simulink model "CBCVacc"  (Simulink 7.5)
settings: Solver=ode4  StartTime=0.0  StopTime=Inf  FixedStep=0.001  RelTol=1e-3
PostLoadFcn:
  | , if any(exist('dsrtsu_mdlpostloadfcn', 'file') == [2, 3, 6]), try dsrtsu_mdlpostloadfcn('Execute', bdroot); catch fprintf('Error in PostLoadFcn (dsrtsu_mdlpostloadfcn) for model "%s":\n %s\n', bdroot, lasterr); end, end,
libraries: simulink x5, rtilib1104 x3, dsparch4 x2
settings Model: DSRTSU_INTERNAL_RTI_VER=380  DSRTSU_INTERNAL_RTI_TYPE=rti1104  Creator=user  LastModifiedBy=user  BufferReuse=off
settings OptimizationCC: BlockReduction=off  ConditionallyExecuteInputs=off  OptimizeBlockIOStorage=off  BufferReuse=off  ExpressionFolding=off  LocalBlockOutputs=off  InitFltsAndDblsToZero=on
settings DebuggingCC: SaveWithParameterizedLinksMsg=none  StrictBusMsg=Warning
settings HardwareCC: ProdIntDivRoundTo=Zero  ProdEndianess=BigEndian  ProdHWDeviceType=Generic->Custom  TargetIntDivRoundTo=Zero  TargetEndianess=BigEndian  TargetHWDeviceType=Generic->Custom
settings RTWCC: SystemTargetFile=rti1104.tlc  MakeCommand=make_rti  TemplateMakefile=rti1104.tmf  Description=dSPACE DS1104 Hardware Platform  ProcessScript=rti1104_make_rtw_hook
settings STFCustomTargetCC: TargetFcnLib=ansi_tfl_tmw.mat  ParMdlRefBuildCompliant=on  GeneratePreprocessorConditionals=Disable all  SystemTargetFile=rti1104.tlc
settings GRTTargetCC: TargetFcnLib=ansi_tfl_tmw.mat  CompOptLevelCompliant=off  MatFileLogging=off  ExtModeMexFile=noextcomm
settings CustomProperty: DataType=RTWOptions_EnumType_C__DSpace_matlab_rti1104_tlc_rti1104_1InitialSimState  Value=RUN
settings EnumStrPairs: String=RUN

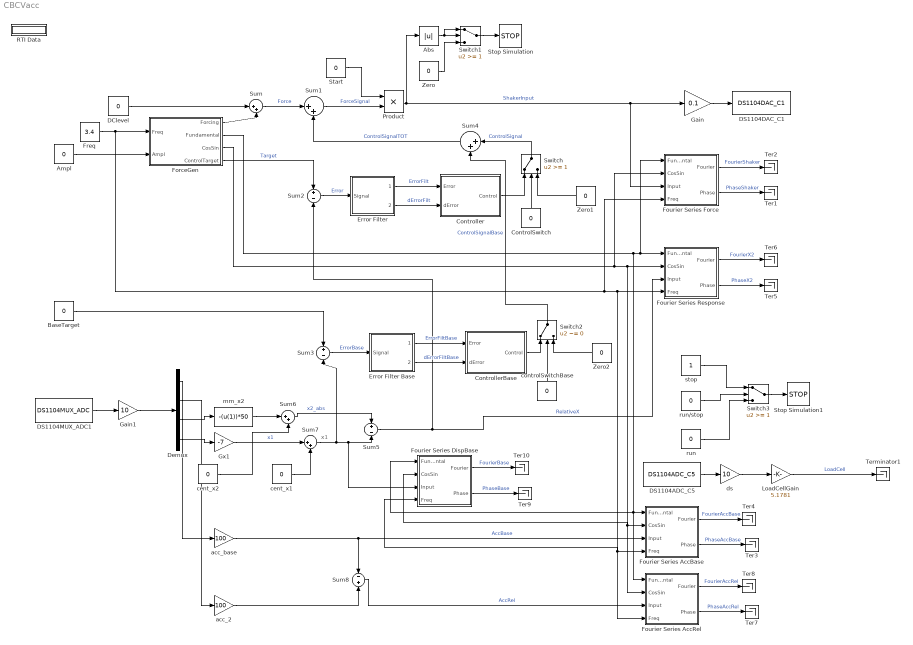
== system CBCVacc ==
  note: x1
  Abs : Abs
  Ampl : Constant  Value=0
  BaseTarget : Constant  Value=0  OutDataType=sfix(16)  OutScaling=2^0
  ControlSwitch : Constant  Value=0  OutDataType=sfix(16)  OutScaling=2^0
  Controller : Subsystem
  ControllerBase : Subsystem
  DClevel : Constant  Value=0  OutDataType=sfix(16)  OutScaling=2^0
  DS1104ADC_C5 : rtilib1104/DS1104 MASTER PPC/DS1104ADC_C5  SystemSampleTime=-1  ChannelNo=5  TriggerMode=0  Reserved1=[]  Reserved2=[]  Reserved3=[]  Reserved4=[]  DialogFcn=gui1104adc  UnitName={ 'DS1104ADC_C' }  UnitValues={ 5 }  DSProperties=struct('RTI',struct('Version',uint32(1),'BlockType',struct('isSLSource',uint8(1),'isSLSink',uint8(0),'isHWSource',uint8(1),'isHWSink',uint8(0),'isSetup',uint8(0),'isInline',uint8(1),'isNonInline',uint8(0),'isInterrupt',uint8(0),'isChannelwise',uint8(1)),'IOBoardType','DS1104MASTER','UnitType','ADC','Identifier','ADC','DialogType','ML','BlockSet','NONE','SlaveProcessor','NONE'))
  DS1104DAC_C1 : rtilib1104/DS1104 MASTER PPC/DS1104DAC_C1  SystemSampleTime=-1  ChannelNo=1  InitValue=0  TermMode=0  TermValue=0  Reserved1=[]  Reserved2=[]  Reserved3=[]  Reserved4=[]  DialogFcn=gui1104dac  UnitName={ 'DS1104DAC_C'}  UnitValues={ 1 }  DSProperties=struct('RTI',struct('Version',uint32(1),'BlockType',struct('isSLSource',uint8(0),'isSLSink',uint8(1),'isHWSource',uint8(0),'isHWSink',uint8(1),'isSetup',uint8(0),'isInline',uint8(1),'isNonInline',uint8(0),'isInterrupt',uint8(0),'isChannelwise',uint8(1)),'IOBoardType','DS1104MASTER','UnitType','DAC','Identifier','DAC','DialogType','ML','BlockSet','NONE','SlaveProcessor','NONE'))
  DS1104MUX_ADC1 : rtilib1104/DS1104 MASTER PPC/DS1104MUX_ADC  SystemSampleTime=-1  ChannelNos=[1 2 3 4]  TriggerMode=0  Reserved1=[]  Reserved2=[]  Reserved3=[]  Reserved4=[]  DialogFcn=gui1104mux_adc  UnitName={ 'DS1104MUX_ADC' }  UnitValues={ [] }  DSProperties=struct('RTI',struct('Version',uint32(1),'BlockType',struct('isSLSource',uint8(1),'isSLSink',uint8(0),'isHWSource',uint8(1),'isHWSink',uint8(0),'isSetup',uint8(0),'isInline',uint8(1),'isNonInline',uint8(0),'isInterrupt',uint8(0),'isChannelwise',uint8(0)),'IOBoardType','DS1104MASTER','UnitType','ADC','Identifier','ADCMUX','DialogType','ML','BlockSet','NONE','SlaveProcessor','NONE'))
  Demux : Demux
  Error Filter : Subsystem
  Error Filter Base : Subsystem
  ForceGen : Subsystem
  Fourier Series AccBase : Subsystem
  Fourier Series AccRel : Subsystem
  Fourier Series DispBase : Subsystem
  Fourier Series Force : Subsystem
  Fourier Series Response : Subsystem
  Freq : Constant  Value=3.4  SampleTime=-1
  Gain : Gain  Gain=0.1
  Gain1 : Gain  Gain=10  ParameterDataType=sfix(16)  ParameterScaling=2^0  OutDataType=sfix(16)  OutScaling=2^0
  Gx1 : Gain  Gain=-7  ParameterDataType=fixdt(1, 16)  ParameterScaling=2^0  OutDataType=fixdt(1, 16)  OutScaling=2^0
  LoadCellGain : Gain  Gain=5.1781  ParameterDataType=fixdt(1, 16)  ParameterScaling=2^0  OutDataType=fixdt(1, 16)  OutScaling=2^0
  Product : Product  OutDataType=sfix(16)  OutScaling=2^0  RndMeth=Zero
  RTI Data : Subsystem  Tag=struct('RTIDataServer',struct('RTIDataServerVs','2','RTIModelDescription','struct(''main'',''CBCVacc'',''sub'','''',''isMp'',0)'))  LoadFcn="if exist('rtidc'), try,  rtidc('DataHostBlockClbLoad', gcbh); catch, disp(['Warning: ''LoadFcn'' for RTI Data block failed: ' lasterr]); end, end,"
      settings: CopyFcn="if exist('rtidc'), try,  rtidc('DataHostBlockClbCopy', gcbh); catch, disp(['Warning: ''CopyFcn'' for RTI Data block failed: ' lasterr]); end, end,"  DeleteFcn="if exist('rtidc'), try,  rtidc('DataHostBlockClbDelete', gcbh); catch, disp(['Warning: ''DeleteFcn'' for RTI Data block failed: ' lasterr]); end, end,"  ModelCloseFcn="if exist('rtidc'), try,  rtidc('DataHostBlockClbModelClose', gcbh); catch, disp(['Warning: ''ModelCloseFcn'' for RTI Data block failed: ' lasterr]); end, end,"  PreSaveFcn="if exist('rtidc'), try,  rtidc('DataHostBlockClbPreSave', gcbh); catch, disp(['Warning: ''PreSaveFcn'' for RTI Data block failed: ' lasterr]); end, end,"  PostSaveFcn="if exist('rtidc'), try,  rtidc('DataHostBlockClbPostSave', gcbh); catch, disp(['Warning: ''PostSaveFcn'' for RTI Data block failed: ' lasterr]); end, end,"  NameChangeFcn="if exist('rtidc'), try,  rtidc('DataHostBlockClbNameChange', gcbh); catch, disp(['Warning: ''NameChangeFcn'' for RTI Data block failed: ' lasterr]); end, end,"
      mask Type: RTI_DATA_HOST
      mask Description:
      | RTI Data Block.
      | This block is used by RTI to store internal model-dependent data.
      | Please keep this block on the root level of the model. Deleting this block will result in data loss.
      | 
      | NEVER DELETE OR COPY THIS BLOCK!
      mask Help:
      | RTI Data Block.
      | This block is used by RTI to store internal model-dependent data.
      | Please keep this block on the root level of the model. Deleting this block will result in data loss.
      | 
      | NEVER DELETE OR COPY THIS BLOCK!
      mask Display:
      | text(0.5, 0.5, 'RTI Data', 'HorizontalAlignment', 'center');
      | plot([1 0]);
  Start : Constant  Value=0  OutDataType=sfix(16)  OutScaling=2^0
  Stop Simulation : Stop
  Stop Simulation1 : Stop
  Sum : Sum  Inputs=|++  OutDataType=sfix(16)  OutScaling=2^0
  Sum1 : Sum  Inputs=|++
  Sum2 : Sum  Inputs=+|-
  Sum3 : Sum  Inputs=+|-
  Sum4 : Sum  Inputs=|++
  Sum5 : Sum  Inputs=+|-
  Sum6 : Sum  Inputs=|++  OutDataType=sfix(16)  OutScaling=2^0
  Sum7 : Sum  Inputs=|++  OutDataType=sfix(16)  OutScaling=2^0
  Sum8 : Sum  Inputs=-|+
  Switch : Switch  Threshold=1
  Switch1 : Switch  Threshold=1
  Switch2 : Switch  Criteria=u2 ~= 0
  Switch3 : Switch  Threshold=1
  Ter{1..10} (10 alike) : Terminator
  Terminator1 : Terminator
  Zero : Constant  Value=0  OutDataType=sfix(16)  OutScaling=2^0
  Zero1 : Constant  Value=0  OutDataType=sfix(16)  OutScaling=2^0
  Zero2 : Constant  Value=0  OutDataType=sfix(16)  OutScaling=2^0
  acc_2 : Gain  Gain=100  ParameterDataType=fixdt(1, 16)  ParameterScaling=2^0  OutDataType=fixdt(1, 16)  OutScaling=2^0
  acc_base : Gain  Gain=100  ParameterDataType=fixdt(1, 16)  ParameterScaling=2^0  OutDataType=fixdt(1, 16)  OutScaling=2^0
  cent_x1 : Constant  Value=0
  cent_x2 : Constant  Value=0
  controlSwitchBase : Constant  Value=0  OutDataType=sfix(16)  OutScaling=2^0
  ds : Gain  Gain=10  ParameterDataType=fixdt(1, 16)  ParameterScaling=2^0  OutDataType=fixdt(1, 16)  OutScaling=2^0
  mm_x2 : Fcn  Expr=-(u(1))*50
  run : Constant  Value=0  OutDataType=sfix(16)  OutScaling=2^0
  run/stop : Constant  Value=0  OutDataType=sfix(16)  OutScaling=2^0
  stop : Constant  OutDataType=sfix(16)  OutScaling=2^0
  wires:
  Freq/1 -> ForceGen/1(Freq), Fourier Series Force/4(Freq), Fourier Series Response/4(Freq), Fourier Series AccBase/4(Freq), Fourier Series AccRel/4(Freq), Fourier Series DispBase/4(Freq)
  Ampl/1 -> ForceGen/2(Ampl)
  ForceGen/3(CosSin) -> Fourier Series Force/2(CosSin), Fourier Series Response/2(CosSin), Fourier Series AccBase/2(CosSin), Fourier Series AccRel/2(CosSin), Fourier Series DispBase/2(CosSin)
  ForceGen/2(Fundamental) -> Fourier Series Response/1(Fundamental), Fourier Series Force/1(Fundamental), Fourier Series AccBase/1(Fundamental), Fourier Series AccRel/1(Fundamental), Fourier Series DispBase/1(Fundamental)
  Fourier Series Response/1(Fourier) -> Ter6/1  "FourierX2"
  Gain/1 -> DS1104DAC_C1/1
  Fourier Series Response/2(Phase) -> Ter5/1  "PhaseX2"
  ForceGen/1(Forcing) -> Sum/2
  DS1104MUX_ADC1/1 -> Gain1/1
  Gain1/1 -> Demux/1
  DClevel/1 -> Sum/1
  Switch1/1 -> Stop Simulation/1
  Abs/1 -> Switch1/2, Switch1/1
  Zero/1 -> Switch1/3
  Start/1 -> Product/1
  Sum/1 -> Sum1/1  "Force"
  Product/1 -> Abs/1, Gain/1, Fourier Series Force/3(Input)  "ShakerInput"
  Error Filter/1(Filtered) -> Controller/1(Error)  "ErrorFilt"
  Error Filter/2(dFiltered) -> Controller/2(dError)  "dErrorFilt"
  Sum2/1 -> Error Filter/1(Signal)  "Error"
  Controller/1(Control) -> Switch/1
  ControlSwitch/1 -> Switch/2
  Zero1/1 -> Switch/3
  ForceGen/4(ControlTarget) -> Sum2/1  "Target"
  Sum1/1 -> Product/2  "ForceSignal"
  Demux/1 -> acc_base/1
  Demux/3 -> mm_x2/1
  Demux/2 -> acc_2/1
  Demux/4 -> Gx1/1
  Error Filter Base/1(Filtered) -> ControllerBase/1(Error)  "ErrorFiltBase"
  Error Filter Base/2(dFiltered) -> ControllerBase/2(dError)  "dErrorFiltBase"
  ControllerBase/1(Control) -> Switch2/1
  Zero2/1 -> Switch2/3
  Sum3/1 -> Error Filter Base/1(Signal)  "ErrorBase"
  BaseTarget/1 -> Sum3/1
  Switch2/1 -> Sum4/2  "ControlSignalBase"
  Sum4/1 -> Sum1/2  "ControlSignalTOT"
  Switch/1 -> Sum4/1  "ControlSignal"
  Fourier Series Force/1(Fourier) -> Ter2/1  "FourierShaker"
  Fourier Series Force/2(Phase) -> Ter1/1  "PhaseShaker"
  Switch3/1 -> Stop Simulation1/1
  run/1 -> Switch3/3
  stop/1 -> Switch3/1
  run/stop/1 -> Switch3/2
  Sum5/1 -> Fourier Series Response/3(Input), Sum2/2  "RelativeX"
  controlSwitchBase/1 -> Switch2/2
  mm_x2/1 -> Sum6/1
  cent_x2/1 -> Sum6/2
  Sum6/1 -> Sum5/1  "x2_abs"
  Gx1/1 -> Sum7/1  "x1"
  cent_x1/1 -> Sum7/2
  Sum7/1 -> Sum3/2, Sum5/2, Fourier Series DispBase/3(Input)
  LoadCellGain/1 -> Terminator1/1  "LoadCell"
  acc_base/1 -> Fourier Series AccBase/3(Input), Sum8/1  "AccBase"
  DS1104ADC_C5/1 -> ds/1
  ds/1 -> LoadCellGain/1
  Fourier Series AccBase/1(Fourier) -> Ter4/1  "FourierAccBase"
  Fourier Series AccBase/2(Phase) -> Ter3/1  "PhaseAccBase"
  Fourier Series AccRel/1(Fourier) -> Ter8/1  "FourierAccRel"
  Fourier Series AccRel/2(Phase) -> Ter7/1  "PhaseAccRel"
  acc_2/1 -> Sum8/2
  Sum8/1 -> Fourier Series AccRel/3(Input)  "AccRel"
  Fourier Series DispBase/1(Fourier) -> Ter10/1  "FourierBase"
  Fourier Series DispBase/2(Phase) -> Ter9/1  "PhaseBase"

== system CBCVacc/Controller ==
  Error : Inport
  dError : Inport  Port=2
  Kd : Constant  Value=0
  Kp : Constant  Value=0
  Product : Product  RndMeth=Zero
  Product1 : Product  RndMeth=Zero
  Sum2 : Sum  Inputs=+|+
  Control : Outport
  wires:
  Kp/1 -> Product/1
  Kd/1 -> Product1/2
  Product/1 -> Sum2/1
  Product1/1 -> Sum2/2
  Error/1 -> Product/2
  Sum2/1 -> Control/1  "Control"
  dError/1 -> Product1/1

== system CBCVacc/ControllerBase ==
  Error : Inport
  dError : Inport  Port=2
  Kd : Constant  Value=0
  Kp : Constant  Value=0
  Product : Product  RndMeth=Zero
  Product1 : Product  RndMeth=Zero
  Sum2 : Sum  Inputs=+|+
  Control : Outport
  wires:
  Kp/1 -> Product/1
  Kd/1 -> Product1/2
  Product/1 -> Sum2/1
  Product1/1 -> Sum2/2
  Error/1 -> Product/2
  Sum2/1 -> Control/1  "Control"
  dError/1 -> Product1/1

== system CBCVacc/Error Filter ==
  Signal : Inport
  Analog Filter Design : dsparch4/Analog Filter Design  method=Butterworth  filttype=Lowpass  N=4  Wlo=2*pi*25  Whi=80  Rp=2  Rs=40
  Sum4 : Sum  Inputs=|-+
  Unit Delay : UnitDelay  SampleTime=-1
  Weighted Sample Time : SampleTimeMath  TsampMathOp=/
  Filtered : Outport
  dFiltered : Outport  Port=2
  wires:
  Unit Delay/1 -> Sum4/1
  Sum4/1 -> Weighted Sample Time/1
  Weighted Sample Time/1 -> dFiltered/1
  Signal/1 -> Analog Filter Design/1
  Analog Filter Design/1 -> Unit Delay/1, Filtered/1, Sum4/2

== system CBCVacc/Error Filter Base ==
  Signal : Inport
  Analog Filter Design : dsparch4/Analog Filter Design  method=Butterworth  filttype=Lowpass  N=4  Wlo=2*pi*25  Whi=80  Rp=2  Rs=40
  Sum4 : Sum  Inputs=|-+
  Unit Delay : UnitDelay  SampleTime=-1
  Weighted Sample Time : SampleTimeMath  TsampMathOp=/
  Filtered : Outport
  dFiltered : Outport  Port=2
  wires:
  Weighted Sample Time/1 -> dFiltered/1
  Analog Filter Design/1 -> Unit Delay/1, Sum4/2, Filtered/1
  Unit Delay/1 -> Sum4/1
  Sum4/1 -> Weighted Sample Time/1
  Signal/1 -> Analog Filter Design/1

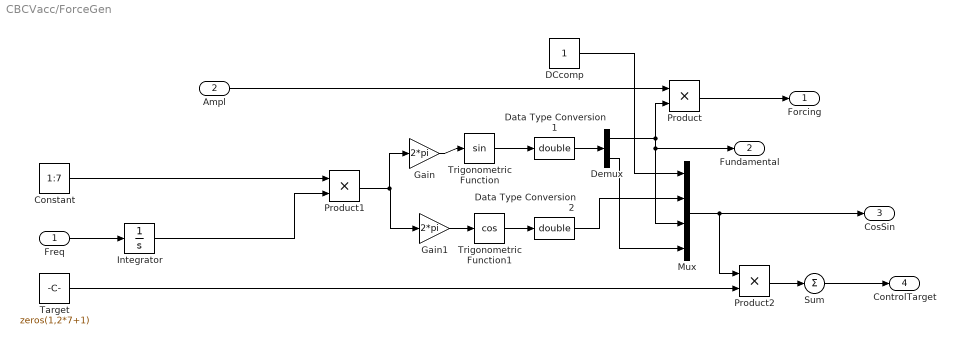
== system CBCVacc/ForceGen ==
  Freq : Inport
  Ampl : Inport  Port=2
  Constant : Constant  Value=1:7
  DCcomp : Constant  OutDataType=sfix(16)  OutScaling=2^0
  Data Type Conversion1 : DataTypeConversion  OutDataTypeMode=double  OutDataTypeStr=double
  Data Type Conversion2 : DataTypeConversion  OutDataTypeMode=double  OutDataTypeStr=double
  Demux : Demux  Outputs=[1,-1]
  Gain : Gain  Gain=2*pi
  Gain1 : Gain  Gain=2*pi
  Integrator : Integrator
  Mux : Mux
  Product : Product
  Product1 : Product
  Product2 : Product  RndMeth=Zero
  Sum : Sum  Inputs=|+|
  Target : Constant  Value=zeros(1,2*7+1)
  Trigonometric Function : Trigonometry
  Trigonometric Function1 : Trigonometry  Operator=cos
  Forcing : Outport
  Fundamental : Outport  Port=2
  CosSin : Outport  Port=3
  ControlTarget : Outport  Port=4
  wires:
  Freq/1 -> Integrator/1
  Trigonometric Function/1 -> Data Type Conversion1/1
  Data Type Conversion1/1 -> Demux/1
  Ampl/1 -> Product/1
  Product/1 -> Forcing/1
  Constant/1 -> Product1/1
  Product1/1 -> Gain/1, Gain1/1
  Trigonometric Function1/1 -> Data Type Conversion2/1
  Mux/1 -> CosSin/1, Product2/1
  Demux/1 -> Product/2, Fundamental/1, Mux/3
  Integrator/1 -> Product1/2
  Gain/1 -> Trigonometric Function/1
  Gain1/1 -> Trigonometric Function1/1
  Demux/2 -> Mux/4
  Data Type Conversion2/1 -> Mux/2
  DCcomp/1 -> Mux/1
  Product2/1 -> Sum/1
  Sum/1 -> ControlTarget/1
  Target/1 -> Product2/2

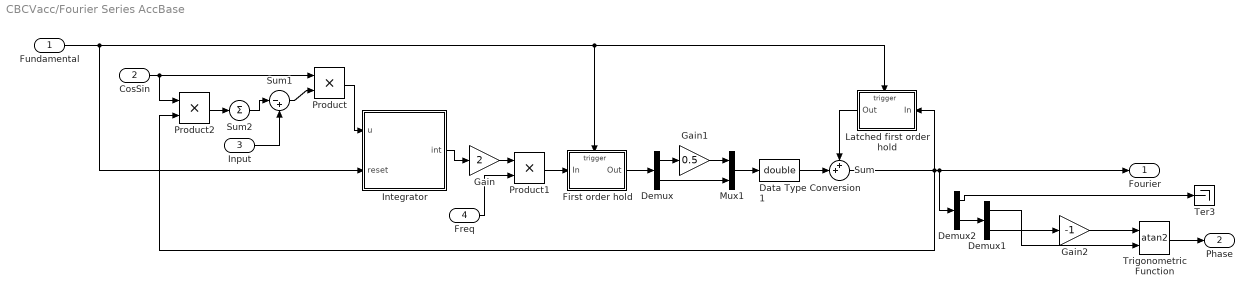
== system CBCVacc/Fourier Series AccBase ==
  Fundamental : Inport
  CosSin : Inport  Port=2
  Input : Inport  Port=3
  Freq : Inport  Port=4
  Data Type Conversion1 : DataTypeConversion  OutDataTypeMode=double  OutDataTypeStr=double
  Demux : Demux  Outputs=[1 -1]
  Demux1 : Demux  Outputs=2
  Demux2 : Demux  Outputs=[1 -1]
  First order hold : Subsystem  TreatAsAtomicUnit=on
  Gain : Gain  Gain=2
  Gain1 : Gain  Gain=0.5
  Gain2 : Gain  Gain=-1
  Integrator : Subsystem
  Latched first order hold : Subsystem  TreatAsAtomicUnit=on
  Mux1 : Mux  Inputs=2
  Product : Product  RndMeth=Zero
  Product1 : Product  RndMeth=Zero
  Product2 : Product  RndMeth=Zero
  Sum : Sum  Inputs=++|
  Sum1 : Sum  Inputs=|-+
  Sum2 : Sum  Inputs=|+|
  Ter3 : Terminator
  Trigonometric Function : Trigonometry  Operator=atan2
  Fourier : Outport
  Phase : Outport  Port=2
  wires:
  Freq/1 -> Product1/2
  Product1/1 -> First order hold/1(In)
  Gain/1 -> Product1/1
  Fundamental/1 -> Integrator/2(reset), First order hold/Trigger, Latched first order hold/Trigger
  Integrator/1(int) -> Gain/1
  Demux/1 -> Gain1/1
  Gain1/1 -> Mux1/1
  Demux/2 -> Mux1/2
  First order hold/1(Out) -> Demux/1
  Mux1/1 -> Data Type Conversion1/1
  Data Type Conversion1/1 -> Sum/2
  Sum/1 -> Product2/2, Latched first order hold/1(In), Fourier/1, Demux2/1
  Latched first order hold/1(Out) -> Sum/1
  Sum1/1 -> Product/2
  Product2/1 -> Sum2/1
  Input/1 -> Sum1/2
  CosSin/1 -> Product/1, Product2/1
  Sum2/1 -> Sum1/1
  Trigonometric Function/1 -> Phase/1
  Product/1 -> Integrator/1(u)
  Demux1/1 -> Trigonometric Function/2
  Demux1/2 -> Gain2/1
  Gain2/1 -> Trigonometric Function/1
  Demux2/2 -> Demux1/1
  Demux2/1 -> Ter3/1

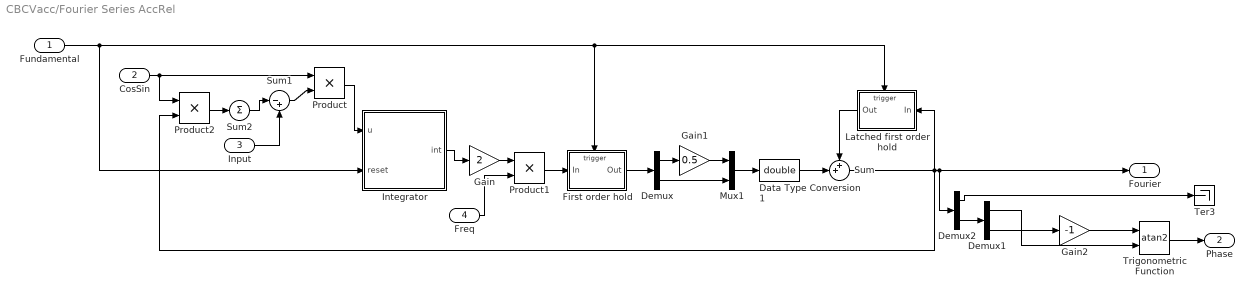
== system CBCVacc/Fourier Series AccRel ==
  Fundamental : Inport
  CosSin : Inport  Port=2
  Input : Inport  Port=3
  Freq : Inport  Port=4
  Data Type Conversion1 : DataTypeConversion  OutDataTypeMode=double  OutDataTypeStr=double
  Demux : Demux  Outputs=[1 -1]
  Demux1 : Demux  Outputs=2
  Demux2 : Demux  Outputs=[1 -1]
  First order hold : Subsystem  TreatAsAtomicUnit=on
  Gain : Gain  Gain=2
  Gain1 : Gain  Gain=0.5
  Gain2 : Gain  Gain=-1
  Integrator : Subsystem
  Latched first order hold : Subsystem  TreatAsAtomicUnit=on
  Mux1 : Mux  Inputs=2
  Product : Product  RndMeth=Zero
  Product1 : Product  RndMeth=Zero
  Product2 : Product  RndMeth=Zero
  Sum : Sum  Inputs=++|
  Sum1 : Sum  Inputs=|-+
  Sum2 : Sum  Inputs=|+|
  Ter3 : Terminator
  Trigonometric Function : Trigonometry  Operator=atan2
  Fourier : Outport
  Phase : Outport  Port=2
  wires:
  Freq/1 -> Product1/2
  Product1/1 -> First order hold/1(In)
  Gain/1 -> Product1/1
  Fundamental/1 -> Integrator/2(reset), First order hold/Trigger, Latched first order hold/Trigger
  Integrator/1(int) -> Gain/1
  Demux/1 -> Gain1/1
  Gain1/1 -> Mux1/1
  Demux/2 -> Mux1/2
  First order hold/1(Out) -> Demux/1
  Mux1/1 -> Data Type Conversion1/1
  Data Type Conversion1/1 -> Sum/2
  Sum/1 -> Product2/2, Latched first order hold/1(In), Fourier/1, Demux2/1
  Latched first order hold/1(Out) -> Sum/1
  Sum1/1 -> Product/2
  Product2/1 -> Sum2/1
  Input/1 -> Sum1/2
  CosSin/1 -> Product/1, Product2/1
  Sum2/1 -> Sum1/1
  Trigonometric Function/1 -> Phase/1
  Product/1 -> Integrator/1(u)
  Demux1/1 -> Trigonometric Function/2
  Demux1/2 -> Gain2/1
  Gain2/1 -> Trigonometric Function/1
  Demux2/2 -> Demux1/1
  Demux2/1 -> Ter3/1

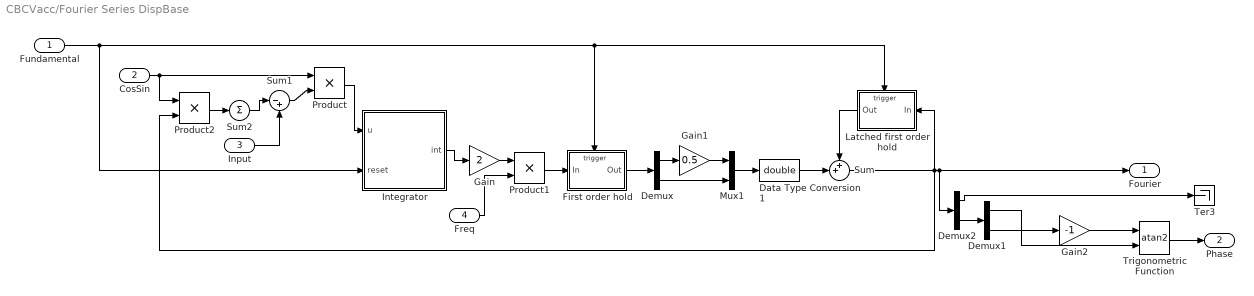
== system CBCVacc/Fourier Series DispBase ==
  Fundamental : Inport
  CosSin : Inport  Port=2
  Input : Inport  Port=3
  Freq : Inport  Port=4
  Data Type Conversion1 : DataTypeConversion  OutDataTypeMode=double  OutDataTypeStr=double
  Demux : Demux  Outputs=[1 -1]
  Demux1 : Demux  Outputs=2
  Demux2 : Demux  Outputs=[1 -1]
  First order hold : Subsystem  TreatAsAtomicUnit=on
  Gain : Gain  Gain=2
  Gain1 : Gain  Gain=0.5
  Gain2 : Gain  Gain=-1
  Integrator : Subsystem
  Latched first order hold : Subsystem  TreatAsAtomicUnit=on
  Mux1 : Mux  Inputs=2
  Product : Product  RndMeth=Zero
  Product1 : Product  RndMeth=Zero
  Product2 : Product  RndMeth=Zero
  Sum : Sum  Inputs=++|
  Sum1 : Sum  Inputs=|-+
  Sum2 : Sum  Inputs=|+|
  Ter3 : Terminator
  Trigonometric Function : Trigonometry  Operator=atan2
  Fourier : Outport
  Phase : Outport  Port=2
  wires:
  Freq/1 -> Product1/2
  Product1/1 -> First order hold/1(In)
  Gain/1 -> Product1/1
  Fundamental/1 -> Integrator/2(reset), First order hold/Trigger, Latched first order hold/Trigger
  Integrator/1(int) -> Gain/1
  Demux/1 -> Gain1/1
  Gain1/1 -> Mux1/1
  Demux/2 -> Mux1/2
  First order hold/1(Out) -> Demux/1
  Mux1/1 -> Data Type Conversion1/1
  Data Type Conversion1/1 -> Sum/2
  Sum/1 -> Product2/2, Latched first order hold/1(In), Fourier/1, Demux2/1
  Latched first order hold/1(Out) -> Sum/1
  Sum1/1 -> Product/2
  Product2/1 -> Sum2/1
  Input/1 -> Sum1/2
  CosSin/1 -> Product/1, Product2/1
  Sum2/1 -> Sum1/1
  Trigonometric Function/1 -> Phase/1
  Product/1 -> Integrator/1(u)
  Demux1/1 -> Trigonometric Function/2
  Demux1/2 -> Gain2/1
  Gain2/1 -> Trigonometric Function/1
  Demux2/2 -> Demux1/1
  Demux2/1 -> Ter3/1

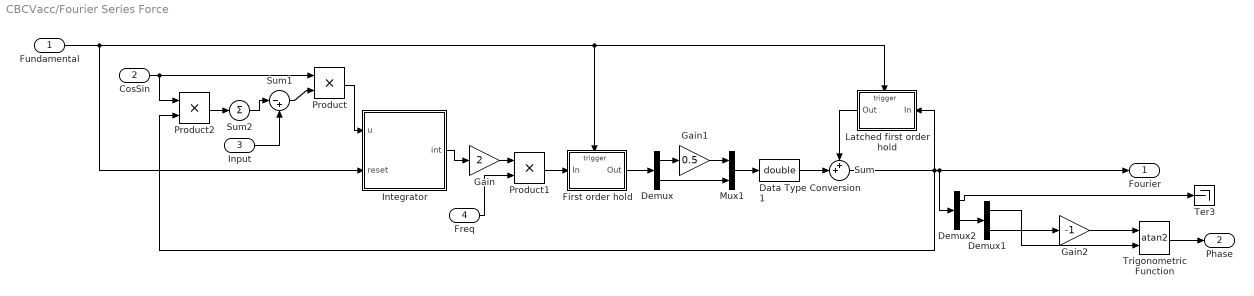
== system CBCVacc/Fourier Series Force ==
  Fundamental : Inport
  CosSin : Inport  Port=2
  Input : Inport  Port=3
  Freq : Inport  Port=4
  Data Type Conversion1 : DataTypeConversion  OutDataTypeMode=double  OutDataTypeStr=double
  Demux : Demux  Outputs=[1 -1]
  Demux1 : Demux  Outputs=2
  Demux2 : Demux  Outputs=[1 -1]
  First order hold : Subsystem  TreatAsAtomicUnit=on
  Gain : Gain  Gain=2
  Gain1 : Gain  Gain=0.5
  Gain2 : Gain  Gain=-1
  Integrator : Subsystem
  Latched first order hold : Subsystem  TreatAsAtomicUnit=on
  Mux1 : Mux  Inputs=2
  Product : Product  RndMeth=Zero
  Product1 : Product  RndMeth=Zero
  Product2 : Product  RndMeth=Zero
  Sum : Sum  Inputs=++|
  Sum1 : Sum  Inputs=|-+
  Sum2 : Sum  Inputs=|+|
  Ter3 : Terminator
  Trigonometric Function : Trigonometry  Operator=atan2
  Fourier : Outport
  Phase : Outport  Port=2
  wires:
  Freq/1 -> Product1/2
  Product1/1 -> First order hold/1(In)
  Gain/1 -> Product1/1
  Fundamental/1 -> Integrator/2(reset), First order hold/Trigger, Latched first order hold/Trigger
  Integrator/1(int) -> Gain/1
  Demux/1 -> Gain1/1
  Gain1/1 -> Mux1/1
  Demux/2 -> Mux1/2
  First order hold/1(Out) -> Demux/1
  Mux1/1 -> Data Type Conversion1/1
  Data Type Conversion1/1 -> Sum/2
  Sum/1 -> Product2/2, Latched first order hold/1(In), Fourier/1, Demux2/1
  Latched first order hold/1(Out) -> Sum/1
  Sum1/1 -> Product/2
  Product2/1 -> Sum2/1
  Input/1 -> Sum1/2
  CosSin/1 -> Product/1, Product2/1
  Sum2/1 -> Sum1/1
  Trigonometric Function/1 -> Phase/1
  Product/1 -> Integrator/1(u)
  Demux1/1 -> Trigonometric Function/2
  Demux1/2 -> Gain2/1
  Gain2/1 -> Trigonometric Function/1
  Demux2/2 -> Demux1/1
  Demux2/1 -> Ter3/1

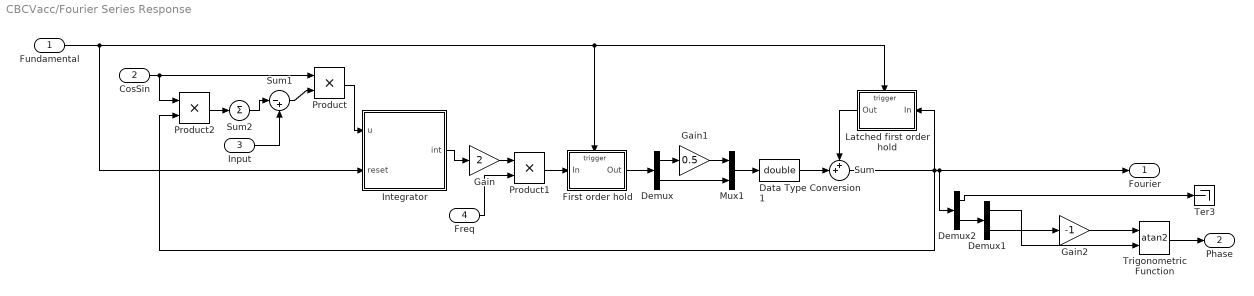
== system CBCVacc/Fourier Series Response ==
  Fundamental : Inport
  CosSin : Inport  Port=2
  Input : Inport  Port=3
  Freq : Inport  Port=4
  Data Type Conversion1 : DataTypeConversion  OutDataTypeMode=double  OutDataTypeStr=double
  Demux : Demux  Outputs=[1 -1]
  Demux1 : Demux  Outputs=2
  Demux2 : Demux  Outputs=[1 -1]
  First order hold : Subsystem  TreatAsAtomicUnit=on
  Gain : Gain  Gain=2
  Gain1 : Gain  Gain=0.5
  Gain2 : Gain  Gain=-1
  Integrator : Subsystem
  Latched first order hold : Subsystem  TreatAsAtomicUnit=on
  Mux1 : Mux  Inputs=2
  Product : Product  RndMeth=Zero
  Product1 : Product  RndMeth=Zero
  Product2 : Product  RndMeth=Zero
  Sum : Sum  Inputs=++|
  Sum1 : Sum  Inputs=|-+
  Sum2 : Sum  Inputs=|+|
  Ter3 : Terminator
  Trigonometric Function : Trigonometry  Operator=atan2
  Fourier : Outport
  Phase : Outport  Port=2
  wires:
  Freq/1 -> Product1/2
  Product1/1 -> First order hold/1(In)
  Gain/1 -> Product1/1
  Fundamental/1 -> Integrator/2(reset), First order hold/Trigger, Latched first order hold/Trigger
  Integrator/1(int) -> Gain/1
  Demux/1 -> Gain1/1
  Gain1/1 -> Mux1/1
  Demux/2 -> Mux1/2
  First order hold/1(Out) -> Demux/1
  Mux1/1 -> Data Type Conversion1/1
  Data Type Conversion1/1 -> Sum/2
  Sum/1 -> Product2/2, Latched first order hold/1(In), Fourier/1, Demux2/1
  Latched first order hold/1(Out) -> Sum/1
  Sum1/1 -> Product/2
  Product2/1 -> Sum2/1
  Input/1 -> Sum1/2
  CosSin/1 -> Product/1, Product2/1
  Sum2/1 -> Sum1/1
  Trigonometric Function/1 -> Phase/1
  Product/1 -> Integrator/1(u)
  Demux1/1 -> Trigonometric Function/2
  Demux1/2 -> Gain2/1
  Gain2/1 -> Trigonometric Function/1
  Demux2/2 -> Demux1/1
  Demux2/1 -> Ter3/1

== system CBCVacc/RTI Data ==
  RTI Data Store : Subsystem  Tag="struct('private',struct('version',struct('dsVer',uint32(2),'dsVerCreation',uint32(2),'RTI',struct('ver','5.3.5','type','RTI1104')),'access',struct('type','Model','isPerm',1,'created',['23-Oct-2012 13:16:32'],'modified',['15-Apr-2015 15:25:54'],'location','')),'public',struct('main',struct('data',[]),'sub',struct('name',{{'CBCVacc'}},'data',{{struct('TH',struct('thTaskInfo',struct('taskType',{'TIMER','HWINT','TMRINT','SWINT'},'tasksNumOf',{1,0,0,0},'srcIds',{{'TIMERA'},{},{},{}},'taskNames',{{['Timer Task 1']},{},{},{}})),'th_tc',struct('dataType','TASK','taskGroupId','','taskGroupList',{{}},'taskSchedulingPolicy','FCFS','taskType','TIMER','blkh',-1,'srcId','TIMERA','srcSgnName',['Timer A interrupt'],'srcCpuName','','taskName',['Timer Task 1  [0.001] s'],'taskNameDisplayExt','','smplTime',0.001,'smplTimeOffs',0,'hasFixedPriority',0,'priority',1,'hasFixedOvc',0,'ovcType',1,'ovcMax',1),'tc_th',struct('dataType','TASK','taskGroupId','','taskGroupList',{{}},'taskSchedulingPolicy','FCFS','taskType','TIMER','blkh',-1,'srcId','TIMERA','srcSgnName',['Timer A interrupt'],'srcCpuName','','taskName',['Timer Task 1  [0.001] s'],'taskNameDisplayExt','','smplTime',0.001,'smplTimeOffs',0,'hasFixedPriority',0,'priority',1,'hasFixedOvc',0,'ovcType',1,'ovcMax',1))}})))"
      mask Type: RTI_DATA_STORE
      mask Description:
      | RTI Data Store Block. This block is used by RTI to store internal model dependent data. Deleting this block will result in data loss.
      | 
      | NEVER DELETE, COPY, OR MODIFY THIS BLOCK!
      mask Help:
      | RTI Data Store Block. This block is used by RTI to store internal model dependent data. Deleting this block will result in data loss.
      | 
      | NEVER DELETE, COPY, OR MODIFY THIS BLOCK!
      mask Display: text(0.5, 0.5, ' ', 'HorizontalAlignment', 'center');

== system CBCVacc/Fourier Series AccBase/First order hold ==
  In : Inport  LatchByDelayingOutsideSignal=on
  Trigger : TriggerPort
  Out : Outport
  wires:
  In/1 -> Out/1

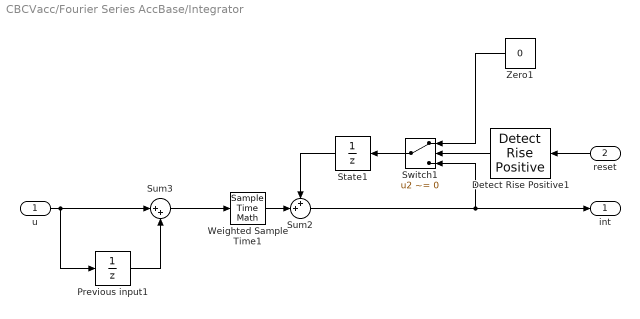
== system CBCVacc/Fourier Series AccBase/Integrator ==
  u : Inport
  reset : Inport  Port=2
  Detect Rise Positive1 : simulink/Logic and Bit Operations/Detect Rise Positive  SystemSampleTime=-1  vinit=0
  Previous input1 : UnitDelay  SampleTime=-1
  State1 : UnitDelay  SampleTime=-1
  Sum2 : Sum  Inputs=++|
  Sum3 : Sum  Inputs=|++
  Switch1 : Switch  Criteria=u2 ~= 0
  Weighted Sample Time1 : SampleTimeMath  TsampMathOp=*  weightValue=0.5
  Zero1 : Constant  Value=0
  int : Outport
  wires:
  Detect Rise Positive1/1 -> Switch1/2
  Zero1/1 -> Switch1/1
  Switch1/1 -> State1/1
  reset/1 -> Detect Rise Positive1/1
  Previous input1/1 -> Sum3/2
  u/1 -> Previous input1/1, Sum3/1
  Sum3/1 -> Weighted Sample Time1/1
  Weighted Sample Time1/1 -> Sum2/2
  Sum2/1 -> int/1, Switch1/3
  State1/1 -> Sum2/1

== system CBCVacc/Fourier Series AccBase/Latched first order hold ==
  In : Inport  LatchByDelayingOutsideSignal=on
  Trigger : TriggerPort
  Out : Outport
  wires:
  In/1 -> Out/1

== system CBCVacc/Fourier Series AccRel/First order hold ==
  In : Inport  LatchByDelayingOutsideSignal=on
  Trigger : TriggerPort
  Out : Outport
  wires:
  In/1 -> Out/1

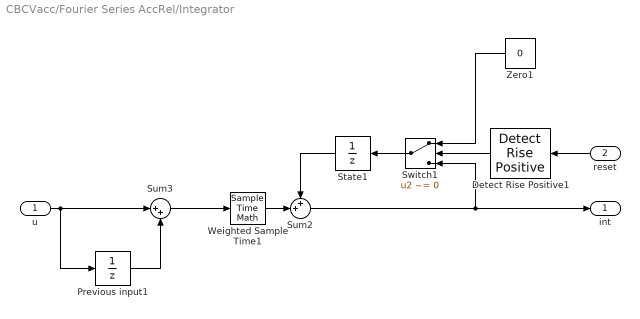
== system CBCVacc/Fourier Series AccRel/Integrator ==
  u : Inport
  reset : Inport  Port=2
  Detect Rise Positive1 : simulink/Logic and Bit Operations/Detect Rise Positive  SystemSampleTime=-1  vinit=0
  Previous input1 : UnitDelay  SampleTime=-1
  State1 : UnitDelay  SampleTime=-1
  Sum2 : Sum  Inputs=++|
  Sum3 : Sum  Inputs=|++
  Switch1 : Switch  Criteria=u2 ~= 0
  Weighted Sample Time1 : SampleTimeMath  TsampMathOp=*  weightValue=0.5
  Zero1 : Constant  Value=0
  int : Outport
  wires:
  Detect Rise Positive1/1 -> Switch1/2
  Zero1/1 -> Switch1/1
  Switch1/1 -> State1/1
  reset/1 -> Detect Rise Positive1/1
  Previous input1/1 -> Sum3/2
  u/1 -> Previous input1/1, Sum3/1
  Sum3/1 -> Weighted Sample Time1/1
  Weighted Sample Time1/1 -> Sum2/2
  Sum2/1 -> int/1, Switch1/3
  State1/1 -> Sum2/1

== system CBCVacc/Fourier Series AccRel/Latched first order hold ==
  In : Inport  LatchByDelayingOutsideSignal=on
  Trigger : TriggerPort
  Out : Outport
  wires:
  In/1 -> Out/1

== system CBCVacc/Fourier Series DispBase/First order hold ==
  In : Inport  LatchByDelayingOutsideSignal=on
  Trigger : TriggerPort
  Out : Outport
  wires:
  In/1 -> Out/1

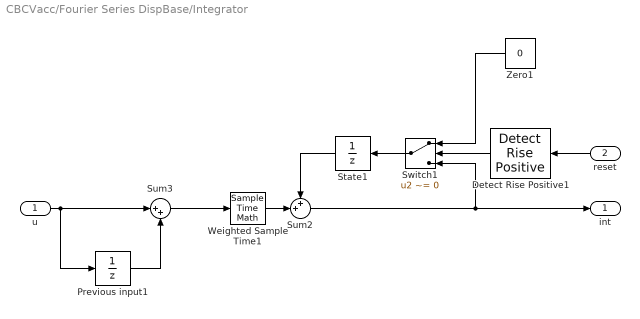
== system CBCVacc/Fourier Series DispBase/Integrator ==
  u : Inport
  reset : Inport  Port=2
  Detect Rise Positive1 : simulink/Logic and Bit Operations/Detect Rise Positive  SystemSampleTime=-1  vinit=0
  Previous input1 : UnitDelay  SampleTime=-1
  State1 : UnitDelay  SampleTime=-1
  Sum2 : Sum  Inputs=++|
  Sum3 : Sum  Inputs=|++
  Switch1 : Switch  Criteria=u2 ~= 0
  Weighted Sample Time1 : SampleTimeMath  TsampMathOp=*  weightValue=0.5
  Zero1 : Constant  Value=0
  int : Outport
  wires:
  Detect Rise Positive1/1 -> Switch1/2
  Zero1/1 -> Switch1/1
  Switch1/1 -> State1/1
  reset/1 -> Detect Rise Positive1/1
  Previous input1/1 -> Sum3/2
  u/1 -> Previous input1/1, Sum3/1
  Sum3/1 -> Weighted Sample Time1/1
  Weighted Sample Time1/1 -> Sum2/2
  Sum2/1 -> int/1, Switch1/3
  State1/1 -> Sum2/1

== system CBCVacc/Fourier Series DispBase/Latched first order hold ==
  In : Inport  LatchByDelayingOutsideSignal=on
  Trigger : TriggerPort
  Out : Outport
  wires:
  In/1 -> Out/1

== system CBCVacc/Fourier Series Force/First order hold ==
  In : Inport  LatchByDelayingOutsideSignal=on
  Trigger : TriggerPort
  Out : Outport
  wires:
  In/1 -> Out/1

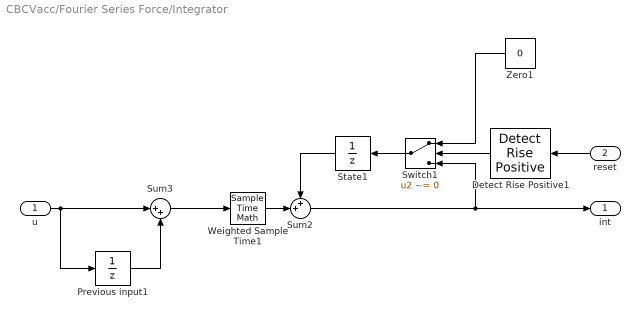
== system CBCVacc/Fourier Series Force/Integrator ==
  u : Inport
  reset : Inport  Port=2
  Detect Rise Positive1 : simulink/Logic and Bit Operations/Detect Rise Positive  SystemSampleTime=-1  vinit=0
  Previous input1 : UnitDelay  SampleTime=-1
  State1 : UnitDelay  SampleTime=-1
  Sum2 : Sum  Inputs=++|
  Sum3 : Sum  Inputs=|++
  Switch1 : Switch  Criteria=u2 ~= 0
  Weighted Sample Time1 : SampleTimeMath  TsampMathOp=*  weightValue=0.5
  Zero1 : Constant  Value=0
  int : Outport
  wires:
  Detect Rise Positive1/1 -> Switch1/2
  Zero1/1 -> Switch1/1
  Switch1/1 -> State1/1
  reset/1 -> Detect Rise Positive1/1
  Previous input1/1 -> Sum3/2
  u/1 -> Previous input1/1, Sum3/1
  Sum3/1 -> Weighted Sample Time1/1
  Weighted Sample Time1/1 -> Sum2/2
  Sum2/1 -> int/1, Switch1/3
  State1/1 -> Sum2/1

== system CBCVacc/Fourier Series Force/Latched first order hold ==
  In : Inport  LatchByDelayingOutsideSignal=on
  Trigger : TriggerPort
  Out : Outport
  wires:
  In/1 -> Out/1

== system CBCVacc/Fourier Series Response/First order hold ==
  In : Inport  LatchByDelayingOutsideSignal=on
  Trigger : TriggerPort
  Out : Outport
  wires:
  In/1 -> Out/1

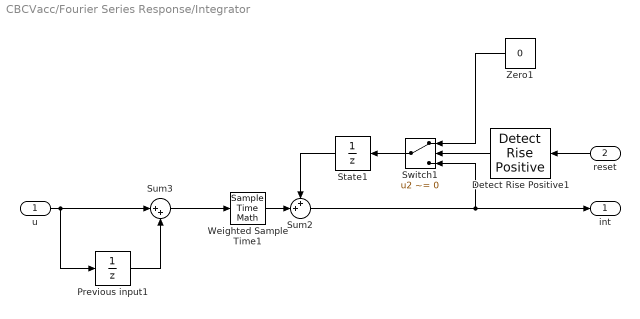
== system CBCVacc/Fourier Series Response/Integrator ==
  u : Inport
  reset : Inport  Port=2
  Detect Rise Positive1 : simulink/Logic and Bit Operations/Detect Rise Positive  SystemSampleTime=-1  vinit=0
  Previous input1 : UnitDelay  SampleTime=-1
  State1 : UnitDelay  SampleTime=-1
  Sum2 : Sum  Inputs=++|
  Sum3 : Sum  Inputs=|++
  Switch1 : Switch  Criteria=u2 ~= 0
  Weighted Sample Time1 : SampleTimeMath  TsampMathOp=*  weightValue=0.5
  Zero1 : Constant  Value=0
  int : Outport
  wires:
  Detect Rise Positive1/1 -> Switch1/2
  Zero1/1 -> Switch1/1
  Switch1/1 -> State1/1
  reset/1 -> Detect Rise Positive1/1
  Previous input1/1 -> Sum3/2
  u/1 -> Previous input1/1, Sum3/1
  Sum3/1 -> Weighted Sample Time1/1
  Weighted Sample Time1/1 -> Sum2/2
  Sum2/1 -> int/1, Switch1/3
  State1/1 -> Sum2/1

== system CBCVacc/Fourier Series Response/Latched first order hold ==
  In : Inport  LatchByDelayingOutsideSignal=on
  Trigger : TriggerPort
  Out : Outport
  wires:
  In/1 -> Out/1

== system CBCVacc/RTI Data/RTI Data Store ==
  RTI Data Store : Subsystem
      mask Type: RTI_DATA_STORE
      mask Description:
      | RTI Data Store Block. This block is used by RTI to store internal model dependent data. Deleting this block will result in data loss.
      | 
      | NEVER DELETE, COPY, OR MODIFY THIS BLOCK!
      mask Help:
      | RTI Data Store Block. This block is used by RTI to store internal model dependent data. Deleting this block will result in data loss.
      | 
      | NEVER DELETE, COPY, OR MODIFY THIS BLOCK!
      mask Display: text(0.5, 0.5, ' ', 'HorizontalAlignment', 'center');

== system CBCVacc/RTI Data/RTI Data Store/RTI Data Store ==
  RTI Data Store : Subsystem
      mask Type: RTI_DATA_STORE
      mask Description:
      | RTI Data Store Block. This block is used by RTI to store internal model dependent data. Deleting this block will result in data loss.
      | 
      | NEVER DELETE, COPY, OR MODIFY THIS BLOCK!
      mask Help:
      | RTI Data Store Block. This block is used by RTI to store internal model dependent data. Deleting this block will result in data loss.
      | 
      | NEVER DELETE, COPY, OR MODIFY THIS BLOCK!
      mask Display: text(0.5, 0.5, ' ', 'HorizontalAlignment', 'center');

== system CBCVacc/RTI Data/RTI Data Store/RTI Data Store/RTI Data Store ==
  RTI Data Store : Subsystem
      mask Type: RTI_DATA_STORE
      mask Description:
      | RTI Data Store Block. This block is used by RTI to store internal model dependent data. Deleting this block will result in data loss.
      | 
      | NEVER DELETE, COPY, OR MODIFY THIS BLOCK!
      mask Help:
      | RTI Data Store Block. This block is used by RTI to store internal model dependent data. Deleting this block will result in data loss.
      | 
      | NEVER DELETE, COPY, OR MODIFY THIS BLOCK!
      mask Display: text(0.5, 0.5, ' ', 'HorizontalAlignment', 'center');

== system CBCVacc/RTI Data/RTI Data Store/RTI Data Store/RTI Data Store/RTI Data Store ==
